simulink model "Actuator_FO_TestBed"  (R2019b)
settings: Solver=ode4  StartTime=0.0  StopTime=10  FixedStep=0.2  RelTol=1e-3  EnableMultiTasking=on
undefined symbols (not defined in the file): MWS
libraries: Lib_Cntrl_FirstOrderActuator_TMATS x1
settings Model: Creator=jwchapm2  LastModifiedBy=bhisma
settings DataIOCC: LimitDataPoints=on  SaveFormat=Array  ReturnWorkspaceOutputs=off
settings OptimizationCC: ExpressionDepthLimit=2147483647  LifeSpan=inf
settings DebuggingCC: UnderspecifiedInitializationDetection=Classic  MergeDetectMultiDrivingBlocksExec=none  SolverPrmCheckMsg=warning  StateNameClashWarn=warning  SFUnexpectedBacktrackingDiag=warning  SFNoUnconditionalDefaultTransitionDiag=warning  SFExecutionAtInitializationDiag=none  ArithmeticOperatorsInVariantConditions=warning
settings HardwareCC: ProdBitPerPointer=32  ProdBitPerSizeT=32  ProdBitPerPtrDiffT=32  ProdLargestAtomicFloat=None  ProdIntDivRoundTo=Undefined  ProdEndianess=Unspecified  ProdWordSize=32  ProdHWDeviceType=32-bit Generic
settings ModelReferenceCC: PropagateSignalLabelsOutOfModel=off
settings SFSimCC: SimUseLocalCustomCode=off  CustomCodeUndefinedFunction=UseInterfaceOnly
settings RTWCC: RTWUseLocalCustomCode=off
settings CodeAppCC: StateflowObjectComments=on
settings GRTTargetCC: TargetLangStandard=C89/C90 (ANSI)  GeneratePreprocessorConditionals=Disable all
settings ConfigComp: CovMetricSettings=dw  CovHtmlReporting=on  CovSaveCumulativeToWorkspaceVar=on  CovSaveSingleToWorkspaceVar=on  CovExternalEMLEnable=off

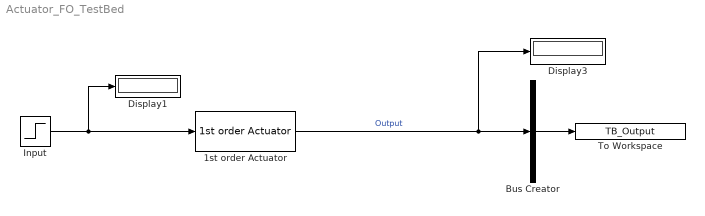
== system Actuator_FO_TestBed ==
  1st order Actuator : Lib_Cntrl_FirstOrderActuator_TMATS/1st order Actuator  Gain_M=MWS.Actuator_FO.Gain  Tau_M=MWS.Actuator_FO.Tau  IC_M=0  MaxSat_M=MWS.Actuator_FO.max  MinSat_M=MWS.Actuator_FO.min  deadband_M=MWS.Actuator_FO.DeadBand  rateLimit_M=MWS.Actuator_FO.RateLim
  Bus Creator : BusCreator  Inputs=1
  Display1 : Display
  Display3 : Display
  Input : Step  Time=MWS.Actuator_FO.Step_Time  Before=MWS.Actuator_FO.Step_IV  After=MWS.Actuator_FO.Inp  SampleTime=0
  To Workspace : ToWorkspace  VariableName=TB_Output  SampleTime=-1
  wires:
  1st order Actuator/1 -> Display3/1, Bus Creator/1  "Output"
  Bus Creator/1 -> To Workspace/1
  Input/1 -> 1st order Actuator/1, Display1/1
